simulink model "t3_5"  (R2017b)
settings: Solver=VariableStepAuto  StartTime=0.0  StopTime=10.0  RelTol=1e-3
settings Model: Creator=zxy19  LastModifiedBy=zxy19

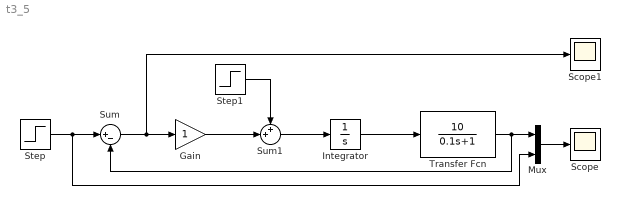
== system t3_5 ==
  Gain : Gain
  Integrator : Integrator
  Mux : Mux  Inputs=2
  Scope : Scope
  Scope1 : Scope
  Step : Step  SampleTime=0
  Step1 : Step  After=0.1  SampleTime=0
  Sum : Sum  Inputs=|+-
  Sum1 : Sum  Inputs=++|
  Transfer Fcn : TransferFcn  Numerator=[10]  Denominator=[0.1 1]
  wires:
  Step/1 -> Mux/2, Sum/1
  Sum/1 -> Scope1/1, Gain/1
  Gain/1 -> Sum1/2
  Step1/1 -> Sum1/1
  Sum1/1 -> Integrator/1
  Integrator/1 -> Transfer Fcn/1
  Mux/1 -> Scope/1
  Transfer Fcn/1 -> Sum/2, Mux/1
